simulink model "robot_pid_cascade"  (R2024b)
settings: Solver=VariableStepAuto  StartTime=0.0  StopTime=10.0  RelTol=1e-3
model workspace (MAT data in the model file):
  pitchd = Simulink.Parameter
  pitchd.Value = 1
  pitchd.Complexity = 'real'
  pitchd.Dimensions = [1 1]
  pitchd.DataType = 'auto'
  yawd = Simulink.Parameter
  yawd.Value = 1
  yawd.Complexity = 'real'
  yawd.Dimensions = [1 1]
  yawd.DataType = 'auto'
values from neighbouring files (symbols this model uses):
  A = [0   1.0000        0        0 ... (first row only)    [invgui.m]    (also in p1.m = 14; p2.m = 14; robot.m = [0 1 0 0; robot_cascade.m = [ 0, 1, 0, 0)
  B = [0; 1.8182; 0; 4.5455]    [invgui.m]    (also in p1.m = 18; p2.m = 18; robot.m = B ./ R; robot_cascade.m = B ./ r_wheel)
  C_xt = eye(4)    [robot.m]    (also in robot_cascade.m; robot_linear.m; robot_lqr.m)
  D_xt = [0;0;0;0]    [robot.m]    (also in robot_cascade.m; robot_linear.m; robot_lqr.m)
  Km = 0.212207    [robot.m]    (also in robot_cascade.m = 16.1290322581; robot_linear.m; robot_lqr.m)
  n = 18.75    [robot.m]    (also in robot_cascade.m; robot_linear.m; robot_lqr.m)
  r_wheel = 0.04    [robot_cascade.m]    (also in robot_linear.m; robot_lqr.m)
libraries: cstblocks x8, slpidlib x2
settings Model: Creator=cosr3  LastModifiedBy=cosr3

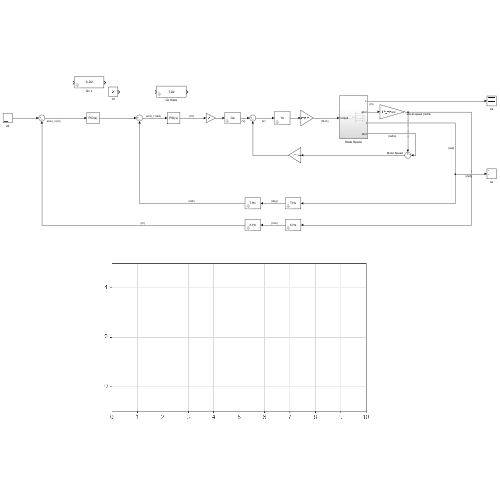
[thumbnail: Simulink's stored preview of the top-level diagram]
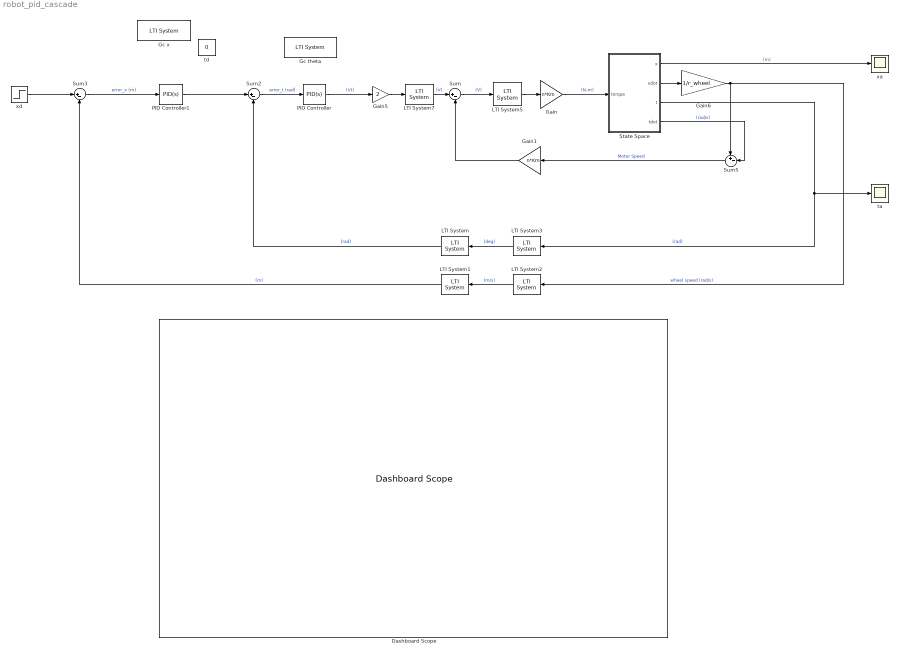
== system robot_pid_cascade ==
  Dashboard Scope : DashboardScope  TimeSpan=10  Ymin=-1  Ymax=5  ScaleAtStop=off
  Gain : Gain  Gain=n*Km
  Gain1 : Gain  Gain=n*Km
  Gain5 : Gain  Gain=2
  Gain6 : Gain  Gain=1/r_wheel
  Gc theta : cstblocks/LTI System  sys=T.D2  IC=[]  PadeOrder=0
  Gc x : cstblocks/LTI System  sys=X.D2  IC=[]  PadeOrder=0
  LTI System : cstblocks/LTI System  sys=T.Hc  IC=[]  PadeOrder=0
  LTI System1 : cstblocks/LTI System  sys=X.Hc  IC=[]  PadeOrder=0
  LTI System2 : cstblocks/LTI System  sys=X.Hs  IC=[]  PadeOrder=0
  LTI System3 : cstblocks/LTI System  sys=T.Hs  IC=[]  PadeOrder=0
  LTI System5 : cstblocks/LTI System  sys=Ye  IC=[]  PadeOrder=0
  LTI System7 : cstblocks/LTI System  sys=Ga  IC=[]  PadeOrder=0
  PID Controller : slpidlib/PID Controller  Controller=PID  Form=Parallel  TimeDomain=Continuous-time  UseExternalTs=off  SampleTime=0.02  IntegratorMethod=Forward Euler  FilterMethod=Forward Euler  ControllerParametersSource=internal  P=7.08497113431161  I=34251.3807405435  UseKiTs=off  D=-9.34091488828225e-05  UseExternalDerivativeSource=off  N=25911.1268640152  UseFilter=on  TunerSelectOption=Transfer Function Based (PID Tuner App)  InitialConditionSource=internal  InitialConditionForIntegrator=0  InitialConditionForFilter=0  DifferentiatorICPrevScaledInput=0  ExternalReset=none  TrackingMode=off  Kt=1  LimitOutput=off  SatLimitsSource=internal  UpperSaturationLimit=inf  LowerSaturationLimit=-inf  LinearizeAsGain=on  AntiWindupMode=none  Kb=1  LimitIntegrator=off  UpperIntegratorSaturationLimit=inf  LowerIntegratorSaturationLimit=-inf  POutMin=[]  POutMax=[]  IOutMin=[]  IOutMax=[]  DOutMin=[]  DOutMax=[]  NOutMin=[]  NOutMax=[]  SumOutMin=[]  SumOutMax=[]  SaturationOutMin=[]  SaturationOutMax=[]  PParamMin=[]  PParamMax=[]  IParamMin=[]  IParamMax=[]  DParamMin=[]  DParamMax=[]  NParamMin=[]  NParamMax=[]  KbParamMin=[]  KbParamMax=[]  KtParamMin=[]  KtParamMax=[]  KbOutMin=[]  KbOutMax=[]  KtOutMin=[]  KtOutMax=[]  IntegratorOutMin=[]  IntegratorOutMax=[]  FilterOutMin=[]  FilterOutMax=[]  SumI1OutMin=[]  SumI1OutMax=[]  SumI2OutMin=[]  SumI2OutMax=[]  SumI3OutMin=[]  SumI3OutMax=[]  SumI4OutMin=[]  SumI4OutMax=[]  SumDOutMin=[]  SumDOutMax=[]  DifferentiatorOutMin=[]  DifferentiatorOutMax=[]  FilterDiffOutCoefMin=[]  FilterDiffOutCoefMax=[]  ReciprocalOutMin=[]  ReciprocalOutMax=[]  SumDenOutMin=[]  SumDenOutMax=[]  SumNumOutMin=[]  SumNumOutMax=[]  DivideOutMin=[]  DivideOutMax=[]  UdiffTsProdOutMin=[]  UdiffTsProdOutMax=[]  NTsProdOutMin=[]  NTsProdOutMax=[]  UintegralTsProdOutMin=[]  UintegralTsProdOutMax=[]  UngainTsProdOutMin=[]  UngainTsProdOutMax=[]  ClampingZeroOutDataTypeStr=Inherit: Inherit via back propagation  ClampingZeroOutMin=[]  ClampingZeroOutMax=[]  FilterDenConstantOutDataTypeStr=Inherit: Inherit via back propagation  FilterDenConstantOutMin=[]  FilterDenConstantOutMax=[]  PCopyOutDataTypeStr=Inherit: Inherit via back propagation  PCopyOutMin=[]  PCopyOutMax=[]  NCopyOutDataTypeStr=Inherit: Inherit via back propagation  NCopyOutMin=[]  NCopyOutMax=[]  IntegratorContinuousStateAttributes=''  IntegratorStateMustResolveToSignalObject=off  IntegratorRTWStateStorageClass=Auto  FilterContinuousStateAttributes=''  FilterStateMustResolveToSignalObject=off  FilterRTWStateStorageClass=Auto  ParallelPVariant=InternalParameters  IdealPVariant=Disabled  IVariant=InternalParameters  DVariant=InternalParameters  IntegratorVariant=Continuous  SatVariant=Disabled  AWVariant=Passthrough  PCopyVariant=Disabled  TRVariant=Disabled  FdbkBlocksVariant=Forward  IdealPFdbkVariant=Disabled  SatFdbkVariant=Disabled  DerivativeFilterVariant=ContFilter  NVariant=InternalParameters  NCopyVariant=Disabled  FilterICVariant=InternalICsFilter  IntegratorICVariant=InternalICs  ExternalResetVariant=Disabled  TRSumVariant=Passthrough  SumFdbkVariant=Disabled  SumVariant=Sum_PID  TsampFilterVariant=InternalTs  TsampNgainVariant=Passthrough  TsampIntegralVariant=Disabled_SignalSpec  ExternalSaturationOutDataTypeStr=Inherit: Same as second input  DerivativeSourceVariant=ErrorSignal  PreIntVariant=InternalPreInt
  PID Controller1 : slpidlib/PID Controller  Controller=PID  Form=Parallel  TimeDomain=Continuous-time  UseExternalTs=off  SampleTime=-1  IntegratorMethod=Forward Euler  FilterMethod=Forward Euler  ControllerParametersSource=internal  P=10.4456433854765  I=81357.7720408598  UseKiTs=off  D=-1.79995607009744e-05  UseExternalDerivativeSource=off  N=80523.6461658895  UseFilter=on  TunerSelectOption=Transfer Function Based (PID Tuner App)  InitialConditionSource=internal  InitialConditionForIntegrator=0  InitialConditionForFilter=0  DifferentiatorICPrevScaledInput=0  ExternalReset=none  TrackingMode=off  Kt=1  LimitOutput=off  SatLimitsSource=internal  UpperSaturationLimit=inf  LowerSaturationLimit=-inf  LinearizeAsGain=on  AntiWindupMode=none  Kb=1  LimitIntegrator=off  UpperIntegratorSaturationLimit=inf  LowerIntegratorSaturationLimit=-inf  POutMin=[]  POutMax=[]  IOutMin=[]  IOutMax=[]  DOutMin=[]  DOutMax=[]  NOutMin=[]  NOutMax=[]  SumOutMin=[]  SumOutMax=[]  SaturationOutMin=[]  SaturationOutMax=[]  PParamMin=[]  PParamMax=[]  IParamMin=[]  IParamMax=[]  DParamMin=[]  DParamMax=[]  NParamMin=[]  NParamMax=[]  KbParamMin=[]  KbParamMax=[]  KtParamMin=[]  KtParamMax=[]  KbOutMin=[]  KbOutMax=[]  KtOutMin=[]  KtOutMax=[]  IntegratorOutMin=[]  IntegratorOutMax=[]  FilterOutMin=[]  FilterOutMax=[]  SumI1OutMin=[]  SumI1OutMax=[]  SumI2OutMin=[]  SumI2OutMax=[]  SumI3OutMin=[]  SumI3OutMax=[]  SumI4OutMin=[]  SumI4OutMax=[]  SumDOutMin=[]  SumDOutMax=[]  DifferentiatorOutMin=[]  DifferentiatorOutMax=[]  FilterDiffOutCoefMin=[]  FilterDiffOutCoefMax=[]  ReciprocalOutMin=[]  ReciprocalOutMax=[]  SumDenOutMin=[]  SumDenOutMax=[]  SumNumOutMin=[]  SumNumOutMax=[]  DivideOutMin=[]  DivideOutMax=[]  UdiffTsProdOutMin=[]  UdiffTsProdOutMax=[]  NTsProdOutMin=[]  NTsProdOutMax=[]  UintegralTsProdOutMin=[]  UintegralTsProdOutMax=[]  UngainTsProdOutMin=[]  UngainTsProdOutMax=[]  ClampingZeroOutDataTypeStr=Inherit: Inherit via back propagation  ClampingZeroOutMin=[]  ClampingZeroOutMax=[]  FilterDenConstantOutDataTypeStr=Inherit: Inherit via back propagation  FilterDenConstantOutMin=[]  FilterDenConstantOutMax=[]  PCopyOutDataTypeStr=Inherit: Inherit via back propagation  PCopyOutMin=[]  PCopyOutMax=[]  NCopyOutDataTypeStr=Inherit: Inherit via back propagation  NCopyOutMin=[]  NCopyOutMax=[]  IntegratorContinuousStateAttributes=''  IntegratorStateMustResolveToSignalObject=off  IntegratorRTWStateStorageClass=Auto  FilterContinuousStateAttributes=''  FilterStateMustResolveToSignalObject=off  FilterRTWStateStorageClass=Auto  ParallelPVariant=InternalParameters  IdealPVariant=Disabled  IVariant=InternalParameters  DVariant=InternalParameters  IntegratorVariant=Continuous  SatVariant=Disabled  AWVariant=Passthrough  PCopyVariant=Disabled  TRVariant=Disabled  FdbkBlocksVariant=Forward  IdealPFdbkVariant=Disabled  SatFdbkVariant=Disabled  DerivativeFilterVariant=ContFilter  NVariant=InternalParameters  NCopyVariant=Disabled  FilterICVariant=InternalICsFilter  IntegratorICVariant=InternalICs  ExternalResetVariant=Disabled  TRSumVariant=Passthrough  SumFdbkVariant=Disabled  SumVariant=Sum_PID  TsampFilterVariant=InternalTs  TsampNgainVariant=Passthrough  TsampIntegralVariant=Disabled_SignalSpec  ExternalSaturationOutDataTypeStr=Inherit: Same as second input  DerivativeSourceVariant=ErrorSignal  PreIntVariant=InternalPreInt
  State Space : Subsystem
  Sum : Sum  Inputs=|+-
  Sum2 : Sum  Inputs=|+-
  Sum3 : Sum  Inputs=|+-
  Sum5 : Sum  Inputs=+-|
  ta : Scope
  td : Constant  Value=0
  xa : Scope
  xd : Step  SampleTime=0
  wires:
  LTI System5/1 -> Gain/1
  Gain/1 -> State Space/1(torque)  "(N-m)"
  LTI System3/1 -> LTI System/1  "(deg)"
  LTI System2/1 -> LTI System1/1  "(m/s)"
  Sum/1 -> LTI System5/1  "(V)"
  Gain1/1 -> Sum/2
  LTI System7/1 -> Sum/1  "(V)"
  PID Controller/1 -> Gain5/1  "(Vt)"
  Sum3/1 -> PID Controller1/1  "error_x (m)"
  Sum2/1 -> PID Controller/1  "error_t (rad)"
  xd/1 -> Sum3/1
  LTI System/1 -> Sum2/2  "(rad)"
  LTI System1/1 -> Sum3/2  "(m)"
  Gain5/1 -> LTI System7/1
  State Space/3(t) -> LTI System3/1, ta/1  "(rad)"
  State Space/2(xdot) -> Gain6/1
  Sum5/1 -> Gain1/1  "Motor Speed"
  State Space/4(tdot) -> Sum5/2  "(rad/s)"
  Gain6/1 -> LTI System2/1, Sum5/1  "wheel speed (rad/s)"
  State Space/1(x) -> xa/1  "(m)"
  PID Controller1/1 -> Sum2/1

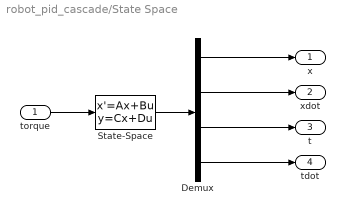
== system robot_pid_cascade/State Space ==
  torque : Inport
  Demux : Demux
  State-Space : StateSpace  A=A  B=B  C=C_xt  D=D_xt  InitialCondition=0
  x : Outport
  xdot : Outport  Port=2
  t : Outport  Port=3
  tdot : Outport  Port=4
  wires:
  Demux/1 -> x/1
  State-Space/1 -> Demux/1
  Demux/4 -> tdot/1
  Demux/2 -> xdot/1
  torque/1 -> State-Space/1
  Demux/3 -> t/1
